simulink model "Host_serial_final_MATLAB"  (Simulink 8.2)
settings: Solver=ode23t  StartTime=0.0  StopTime=10  RelTol=1e-3
InitFcn:
  | tstop = str2num(get_param(bdroot,'StopTime'));
StopFcn:
  | instrreset
undefined symbols (not defined in the file or in its folder): sigbuilder_block
settings Model: Creator=deastman  LastModifiedBy=pvinnako
settings DataIOCC: LimitDataPoints=off  SignalLoggingSaveFormat=Dataset  SaveOutput=off  SaveTime=off
settings DebuggingCC: SolverPrmCheckMsg=none  ParameterOverflowMsg=warning  FcnCallInpInsideContextMsg=EnableAllAsWarning  StrictBusMsg=Warning
settings ConfigurationSet: Description=SimMechanics 2G

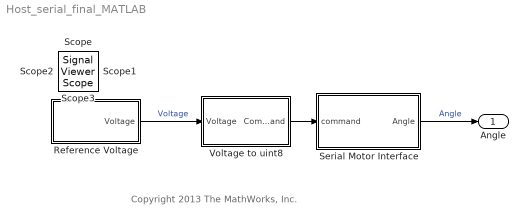
== system Host_serial_final_MATLAB ==
  note: Copyright 2013 The MathWorks, Inc.
  Reference Voltage : Subsystem  Tag=STV Subsys  LoadFcn=sigbuilder_block('load',[6 4.5 466.5 247.5 ]);  StartFcn=sigbuilder_block('start');  StopFcn=sigbuilder_block('stop');  ClipboardFcn=sigbuilder_block('clipboard');  mask(Sigbuilder block){}
      mask help: Sigbuilder GUI
      mask init:
      | if ~strcmp(get_param(bdroot(gcbh),'SimulationStatus'),'stopped') tuvar = sigbuilder_block('maskInit'); end
      settings: CopyFcn=sigbuilder_block('copy');  DeleteFcn=sigbuilder_block('delete');  ModelCloseFcn=sigbuilder_block('modelClose');  PreSaveFcn=sigbuilder_block('preSave');  PauseFcn=sigbuilder_block('pause')  ContinueFcn=sigbuilder_block('continue')  NameChangeFcn=sigbuilder_block('namechange');  OpenFcn=sigbuilder_block('open',[168.75 307.5 810 456 ]);  CloseFcn=sigbuilder_block('close');
      mask Display: plot(0,0,100,100,[10,10,40,40,10],[80,20,20,80,80],[40,10],[50,50], [40,27,10],[65,72,56],[40,25,25,10],[28,28,43,43]);
  Serial Motor Interface : Subsystem  StartFcn=|  StopFcn=|
      StartFcn=|
      | openInstr = instrfind;                           
      | if ~isempty(openInstr)                           
      |   fclose(openInstr);                             
      |   delete(openInstr);                             
      | end                                              
      | clear openInstr                                  
      | s = serial('COM4', 'BaudRate', 9600,'Timeout',5);
      | fopen(s);
      StopFcn=|
      | fclose(s);
      | delete(s);
      | clear s
  Voltage to uint8 : Subsystem
  Angle : Outport
  Scope : SignalViewerScope  IOType=viewer  NumInputPorts=2  RefreshTime=0.035000
      settings: TimeRange=10  YMin=-3~-150  YMax=3~100
  Scope1 : SignalViewerScope  IOType=viewer  NumInputPorts=2  ZoomMode=xonly  RefreshTime=0.035000
      settings: ShowLegends=on  TimeRange=10  YMin=-5~-125  YMax=5~125  SaveName=ScopeData3
  Scope2 : SignalViewerScope  IOType=viewer  RefreshTime=0.035000
  Scope3 : SignalViewerScope  IOType=viewer  RefreshTime=0.035000
      settings: SaveName=ScopeData2
  wires:
  Reference Voltage/1(Voltage) -> Voltage to uint8/1(Voltage)  "Voltage"
  Serial Motor Interface/1(Angle) -> Angle/1  "Angle"
  Voltage to uint8/1(Command) -> Serial Motor Interface/1(command)

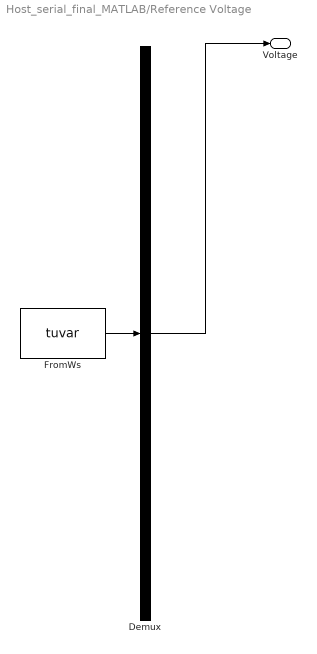
== system Host_serial_final_MATLAB/Reference Voltage ==
  Demux : Demux  Tag=STV Demux  Outputs=1
  FromWs : FromWorkspace  Tag=STV FromWs  VariableName=tuvar  SampleTime=1/100  SigBuilderData=DataTag0  VnvData=DataTag1
      SigBuilderData=|
      | common.afterFinalStr = 'Extrapolate'
      | common.sampleTime = '1/100'
      | dataSet(1).timeRange = [0 10]
      | dataSet(1).name = 'Bounds1'
      | dataSet(2).timeRange = [0 10]
      | dataSet(2).name = 'Bounds5'
      | dataSet(3).timeRange = [0 20]
      | dataSet(3).name = 'Sine3'
      | dataSet(4).timeRange = [0 20]
      | dataSet(4).name = 'Sine5'
      | dataSet(5).timeRange = [0 20]
      | dataSet(5).name = 'Step1'
      | dataSet(6).timeRange = [0 20]
      | dataSet(6).name = 'Step2'
      | dataSet(7).timeRange = [0 10]
      | dataSet(7).name = 'RampSquare'
      | dataSet(8).timeRange = [0 10]
      | dataSet(8).name = 'Steps'
      | dataSet(9).timeRange = [0 10]
      | dataSet(9).name = 'Small Steps'
      | dataSet(10).timeRange = [0 10]
      | dataSet(10).name = 'Square'
      | dataSet(11).timeRange = [0 55]
      | dataSet(11).name = 'DeadZone'
      | sbobj.Groups(1).Name = 'Bounds1'
      | sbobj.Groups(1).Signals.Name = 'Voltage'
      | sbobj.Groups(1).Signals.XData = [0 2.5 2.5 5 5 7.5 7.5 10]
      | sbobj.Groups(1).Signals.YData = [1 1 -1 -1 1 1 -1 -1]
      | sbobj.Groups(2).Name = 'Bounds5'
      | sbobj.Groups(2).Signals.Name = 'Voltage'
      | sbobj.Groups(2).Signals.XData = [0 2.5 2.5 5 5 7.5 7.5 10]
      | sbobj.Groups(2).Signals.YData = [5 5 -5 -5 5 5 -5 -5]
      | sbobj.Groups(3).Name = 'Sine3'
      | sbobj.Groups(3).Signals.Name = 'Voltage'
      | sbobj.Groups(3).Signals.XData = [0 0.01 0.02 0.03 0.04 0.05 0.06 0.07 0.08 0.09 0.1 0.11 ... (2001 elements, 1x2001)]
      | sbobj.Groups(3).Signals.YData = [0 0.0299995000025 0.05999600008 0.0899865006075 0.11996800256 0.149937507812 0.179892019438 0.209828542013 0.239744081908 0.269635647594 0.29950024994 0.329334902512 ... (2001 elements, 1x2001)]
      | sbobj.Groups(3).TimeRange = [0 20]
      | sbobj.Groups(4).Name = 'Sine5'
      | sbobj.Groups(4).Signals.Name = 'Voltage'
      | sbobj.Groups(4).Signals.XData = [0 0.01 0.02 0.03 0.04 0.05 0.06 0.07 0.08 0.09 0.1 0.11 ... (2001 elements, 1x2001)]
      | sbobj.Groups(4).Signals.YData = [0 0.0499991666708 0.0999933334667 0.149977501012 0.199946670933 0.249895846353 0.299820032397 0.349714236688 0.399573469846 0.44939274599 0.499167083234 0.548891504186 ... (2001 elements, 1x2001)]
      | sbobj.Groups(4).TimeRange = [0 20]
      | sbobj.Groups(5).Name = 'Step1'
      | sbobj.Groups(5).Signals.Name = 'Voltage'
      | sbobj.Groups(5).Signals.XData = [0 0.01 0.02 0.03 0.04 0.05 0.06 0.07 0.08 0.09 0.1 0.11 ... (2001 elements, 1x2001)]
      | sbobj.Groups(5).Signals.YData = [0 0 0 0 0 0 0 0 0 0 0 0 ... (2001 elements, 1x2001)]
      | sbobj.Groups(5).TimeRange = [0 20]
      | sbobj.Groups(6).Name = 'Step2'
      | sbobj.Groups(6).Signals.Name = 'Voltage'
      | sbobj.Groups(6).Signals.XData = [0 0.01 0.02 0.03 0.04 0.05 0.06 0.07 0.08 0.09 0.1 0.11 ... (2001 elements, 1x2001)]
      | sbobj.Groups(6).Signals.YData = [0 0 0 0 0 0 0 0 0 0 0 0 ... (2001 elements, 1x2001)]
      | sbobj.Groups(6).TimeRange = [0 20]
      | sbobj.Groups(7).Name = 'RampSquare'
      | sbobj.Groups(7).Signals.Name = 'Voltage'
      | sbobj.Groups(7).Signals.XData = [0 1 1 2 2 3 3 4 4 5 5 6 6 7 7 8 8 9 9 9.8 9.8 10]
      | sbobj.Groups(7).Signals.YData = [0 0.75 0 -0.75 0 1.5 0 -1.5 2 2 -2 -2 3 3 -3 -3 1 1 -1 -1 0 0]
      | sbobj.Groups(8).Name = 'Steps'
      | sbobj.Groups(8).Signals.Name = 'Voltage'
      | sbobj.Groups(8).Signals.XData = [0 1.52 1.52 2.4 2.4 3.66 3.68 4.64 4.64 6.02 6.02 7 7 8.96 8.96 10]
      | sbobj.Groups(8).Signals.YData = [2 2 -3 -3 3 -1 1.95 1.95 -2 -2 0.7 0.7 -1.05 -0.05 0 0]
      | sbobj.Groups(9).Name = 'Small Steps'
      | sbobj.Groups(9).Signals.Name = 'Voltage'
      | sbobj.Groups(9).Signals.XData = [0 0.5 0.5 1.02 1.02 2 2 2.58 2.58 3.78 3.78 4.64 4.64 5.28 5.28 6 6 7 7 9 9 10]
      | sbobj.Groups(9).Signals.YData = [0.4 0.4 0.75 0.75 1.5 3 1.55 1.55 3.55 3.55 -3.05 -3.05 -1 -1 -0.45 -0.45 0.7 0.7 -2.05 -0.05 1 1]
      | sbobj.Groups(10).Name = 'Square'
      | sbobj.Groups(10).Signals.Name = 'Voltage'
      | sbobj.Groups(10).Signals.XData = [0 0.5 0.5 1.02 1.02 1.5 1.5 2 2 2.5 2.5 3 3 4 4 5 5 6 6 7 7 8 8 9 9 9.8 9.8 10]
      | sbobj.Groups(10).Signals.YData = [0.4 0.4 -0.4 -0.4 1 1 -1 -1 1.5 1.5 -1.5 -1.5 2 2 -2 -2 3 3 -3 -3 1.3 1.3 -1.3 -1.3 -4 -4 0 0]
      | sbobj.Groups(11).Name = 'DeadZone'
      | sbobj.Groups(11).Signals.Name = 'Voltage'
      | sbobj.Groups(11).Signals.XData = [0 5 5 10 10 15 15 20 25 30 30 35 40 45 50 50 55]
      | sbobj.Groups(11).Signals.YData = [0 0 0.16 0.16 0.3 0.3 0.7 0.7 -0.205 -0.205 -0.355 -0.35 -0.605 -0.605 0.005 0 0]
      | sbobj.Groups(11).TimeRange = [0 55]
  Voltage : Outport  Tag=STV Outport
  wires:
  Demux/1 -> Voltage/1
  FromWs/1 -> Demux/1

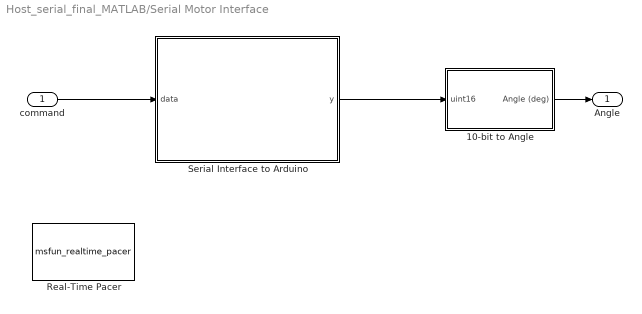
== system Host_serial_final_MATLAB/Serial Motor Interface ==
  command : Inport  OutDataTypeStr=uint8  SampleTime=0.01
  10-bit to Angle : Subsystem
  Real-Time Pacer : M-S-Function  FunctionName=msfun_realtime_pacer  Parameters=simTimePerRealTime  mask(RealTime_Pacer){simTimePerRealTime=1}
      mask prompts: simTimePerRealTime "Speedup (Simulation Time / Real Time):"
      mask help:
      | Slow down a simulation to track real (i.e., wall clock) elapsed time.
      |
      | "Speedup" specifies the ratio between simulation time and real time
      | • Speedup = N => N sec. of simulation time per sec. of real time
      | • Speedup can be fractional (e.g., 0.5, 1.3).
      | • Speedup = inf => allow simulation to run at full speed
      |
      | Click on the Help button for details.
      mask Help: web('realtime_pacer_help.html', '-helpbrowser')
      mask Display: fprintf('Real-Time Pacer\nSpeedup = %g', simTimePerRealTime)
  Serial Interface to Arduino : MATLAB Function  TreatAsAtomicUnit=on  SystemSampleTime=1/100
  Angle : Outport
  wires:
  Serial Interface to Arduino/1(y) -> 10-bit to Angle/1(uint16)
  command/1 -> Serial Interface to Arduino/1(data)
  10-bit to Angle/1(Angle (deg)) -> Angle/1

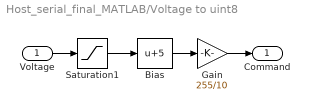
== system Host_serial_final_MATLAB/Voltage to uint8 ==
  Voltage : Inport
  Bias : Bias  Bias=5
  Gain : Gain  Gain=255/10  OutDataTypeStr=uint8
  Saturation1 : Saturate  UpperLimit=5  LowerLimit=-5
  Command : Outport
  wires:
  Bias/1 -> Gain/1
  Saturation1/1 -> Bias/1
  Gain/1 -> Command/1
  Voltage/1 -> Saturation1/1

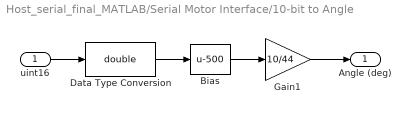
== system Host_serial_final_MATLAB/Serial Motor Interface/10-bit to Angle ==
  uint16 : Inport
  Bias : Bias  Bias=-500
  Data Type Conversion : DataTypeConversion  OutDataTypeStr=double
  Gain1 : Gain  Gain=10/44
  Angle (deg) : Outport
  wires:
  Gain1/1 -> Angle (deg)/1
  uint16/1 -> Data Type Conversion/1
  Data Type Conversion/1 -> Bias/1
  Bias/1 -> Gain1/1

== matlab function Serial Motor Interface/Serial Interface to Arduino ==
  data: data input uint8 size=1; y output int16 size=1
function y = serialFcn(data)

    coder.extrinsic('fread','fwrite','instrfind')
    
    persistent s last
   
    % Declaring parameters
    HEADER = 'A';
    PACKET_SIZE = 4;
    packet = zeros(PACKET_SIZE,1,'int16');
   
    % Initializing the serial object
    if isempty(s)
        s = instrfind;        
        last = int16(0);
    end
    
    % Write data to the serial port  
    fwrite(s,data,'uint8');
    
    % Read data from the serial port
    packet = int16(fread(s, PACKET_SIZE, 'uint8'));
    
    % Check for header and convert two bytes to single int16
    if (packet(1) ~= HEADER)
          y = last;
    else 
          y  = 2^8*packet(3)+packet(2);
          last = y;
    end
% y= 0;
